simulink model "indicator"  (R2020b)
settings: Solver=VariableStepAuto  StartTime=0.0  StopTime=100  RelTol=1e-3
model workspace (MAT data in the model file):
  ind = Simulink.Parameter
  ind.DataType = 'boolean'
  ind.Dimensions = [0 0]
settings Model: PacingRate=0.350000  Creator=Training  LastModifiedBy=Training

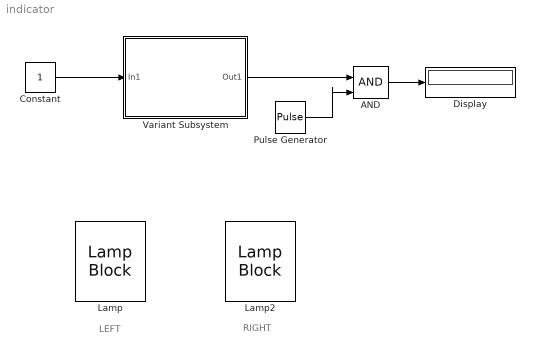
== system indicator ==
  note: LEFT
  note: RIGHT
  AND : Logic  IconShape=distinctive  AllPortsSameDT=off  OutDataTypeStr=boolean
  Constant : Constant
  Display : Display
  Lamp : LampBlock
  Lamp2 : LampBlock
  Pulse Generator : DiscretePulseGenerator  PulseType=Time based  Period=10  PulseWidth=50
  Variant Subsystem : Subsystem  Variant=on
  wires:
  Constant/1 -> Variant Subsystem/1(In1)
  Variant Subsystem/1(Out1) -> AND/1
  Pulse Generator/1 -> AND/2
  AND/1 -> Display/1

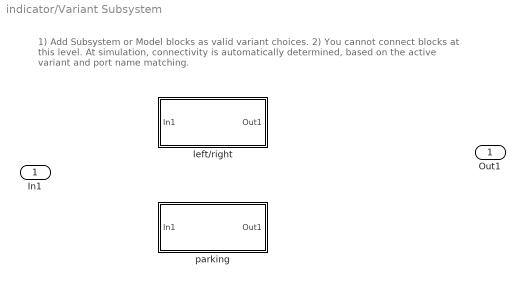
== system indicator/Variant Subsystem ==
  note: 1) Add Subsystem or Model blocks as valid variant choices.
      | 2) You cannot connect blocks at this level. At simulation, connectivity is automatically
      | determined, based on the active variant and port name matching.
  In1 : Inport
  left/right : Subsystem  VariantControl=ind==0
  parking : Subsystem  VariantControl=ind==1
  Out1 : Outport

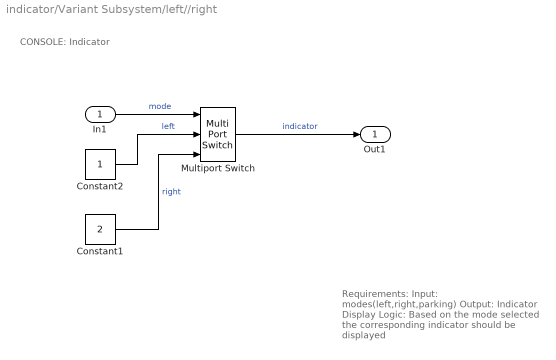
== system indicator/Variant Subsystem/left//right ==
  note: Requirements:
      | Input: modes(left,right,parking)
      | Output: Indicator Display
      | Logic: Based on the mode selected the corresponding indicator should be displayed
  note: CONSOLE: Indicator
  In1 : Inport
  Constant1 : Constant  Value=2
  Constant2 : Constant
  Multiport Switch : MultiPortSwitch  Inputs=2
  Out1 : Outport
  wires:
  In1/1 -> Multiport Switch/1  "mode"
  Constant1/1 -> Multiport Switch/3  "right"
  Constant2/1 -> Multiport Switch/2  "left"
  Multiport Switch/1 -> Out1/1  "indicator"

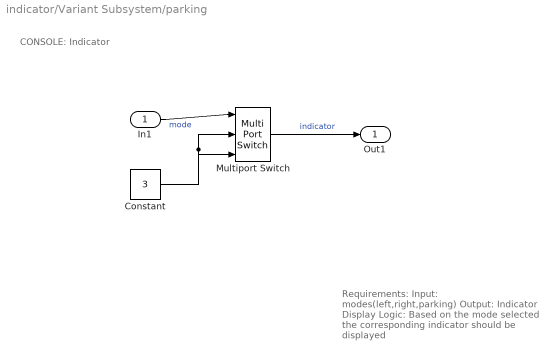
== system indicator/Variant Subsystem/parking ==
  note: Requirements:
      | Input: modes(left,right,parking)
      | Output: Indicator Display
      | Logic: Based on the mode selected the corresponding indicator should be displayed
  note: CONSOLE: Indicator
  In1 : Inport
  Constant : Constant  Value=3
  Multiport Switch : MultiPortSwitch  Inputs=2
  Out1 : Outport
  wires:
  Constant/1 -> Multiport Switch/3, Multiport Switch/2
  In1/1 -> Multiport Switch/1  "mode"
  Multiport Switch/1 -> Out1/1  "indicator"
